simulink model "BMS"  (R2022b)
settings: Solver=VariableStepAuto  StartTime=0.0  StopTime=inf  RelTol=1e-3
libraries: simulink x2
settings Model: PacingRate=0.710000  Creator=admin  LastModifiedBy=DELL

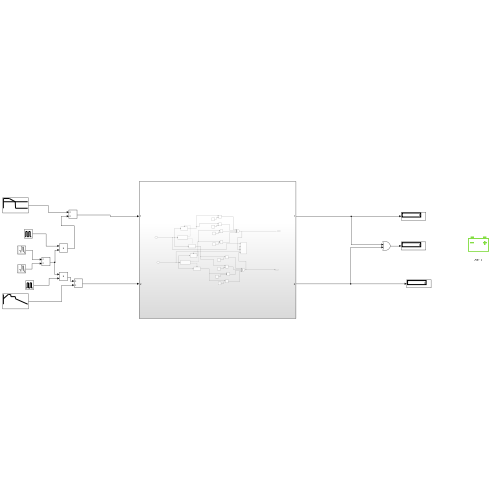
[thumbnail: Simulink's stored preview of the top-level diagram]
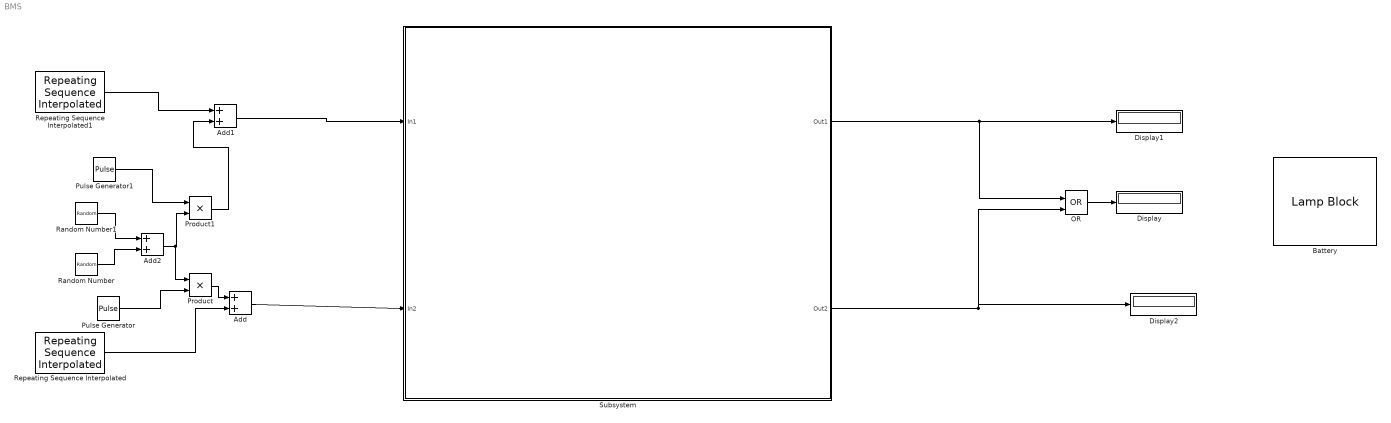
== system BMS ==
  Add : Sum
  Add1 : Sum
  Add2 : Sum
  Battery : LampBlock  LabelPosition=Bottom  Icon=Battery
  Display : Display
  Display1 : Display
  Display2 : Display
  OR : Logic  Operator=OR  IconShape=distinctive  AllPortsSameDT=off  OutDataTypeStr=boolean
  Product : Product
  Product1 : Product
  Pulse Generator : DiscretePulseGenerator  PulseType=Time based  Period=22  PulseWidth=2  PhaseDelay=20
  Pulse Generator1 : DiscretePulseGenerator  PulseType=Time based  Period=37  PulseWidth=2  PhaseDelay=40
  Random Number : RandomNumber  Variance=7  SampleTime=0.1
  Random Number1 : RandomNumber  Mean=-5  Variance=13  SampleTime=0.1
  Repeating Sequence Interpolated : simulink/Sources/Repeating Sequence Interpolated  OutValues=[12.8 14.2 14.2 13.5 13.5 12.8 11].'  TimeValues=[0 0.2 0.30 0.31 0.49 0.50 1].'  LookUpMeth=Interpolation-Use End Values  tsamp=0.01  OutMin=[]  OutMax=[]  OutDataTypeStr=double  OutputDataTypeScalingMode=double  OutDataType=fixdt(0,8)  OutScaling=2^-10
  Repeating Sequence Interpolated1 : simulink/Sources/Repeating Sequence Interpolated  OutValues=[3 3 0 -6 -6].'  TimeValues=[0 0.25 0.49 0.5 1].'  LookUpMeth=Interpolation-Use End Values  tsamp=0.01  OutMin=[]  OutMax=[]  OutDataTypeStr=double  OutputDataTypeScalingMode=double  OutDataType=fixdt(0,8)  OutScaling=2^-10
  Subsystem : Subsystem
  wires:
  Pulse Generator/1 -> Product/2
  Pulse Generator1/1 -> Product1/1
  Random Number/1 -> Add2/2
  Add2/1 -> Product/1, Product1/2
  Random Number1/1 -> Add2/1
  Product1/1 -> Add1/2
  Repeating Sequence Interpolated1/1 -> Add1/1
  Product/1 -> Add/1
  Repeating Sequence Interpolated/1 -> Add/2
  OR/1 -> Display/1
  Add1/1 -> Subsystem/1(In1)
  Add/1 -> Subsystem/2(In2)
  Subsystem/1(Out1) -> OR/1, Display1/1
  Subsystem/2(Out2) -> OR/2, Display2/1

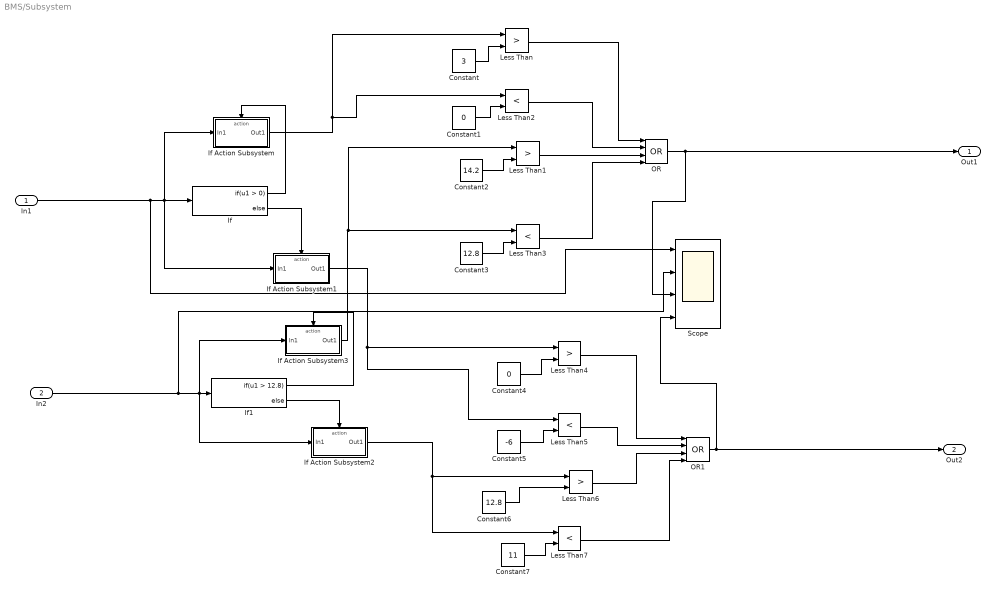
== system BMS/Subsystem ==
  In1 : Inport
  In2 : Inport  Port=2
  Constant : Constant  Value=3
  Constant1 : Constant  Value=0
  Constant2 : Constant  Value=14.2
  Constant3 : Constant  Value=12.8
  Constant4 : Constant  Value=0
  Constant5 : Constant  Value=-6
  Constant6 : Constant  Value=12.8
  Constant7 : Constant  Value=11
  If : If
  If Action Subsystem : Subsystem  TreatAsAtomicUnit=on
  If Action Subsystem1 : Subsystem  TreatAsAtomicUnit=on
  If Action Subsystem2 : Subsystem  TreatAsAtomicUnit=on
  If Action Subsystem3 : Subsystem  TreatAsAtomicUnit=on
  If1 : If  IfExpression=u1 > 12.8
  Less Than{,1,4,6} (4 alike) : RelationalOperator  Operator=>  OutDataTypeStr=boolean  RndMeth=Simplest  InputSameDT=off
  Less Than{2..3,5,7} (4 alike) : RelationalOperator  Operator=<  OutDataTypeStr=boolean  RndMeth=Simplest  InputSameDT=off
  OR : Logic  Operator=OR  Inputs=4  IconShape=distinctive  AllPortsSameDT=off  OutDataTypeStr=boolean
  OR1 : Logic  Operator=OR  Inputs=4  IconShape=distinctive  AllPortsSameDT=off  OutDataTypeStr=boolean
  Scope : Scope  NumInputPorts=4
  Out1 : Outport
  Out2 : Outport  Port=2
  wires:
  Constant4/1 -> Less Than4/2
  Constant6/1 -> Less Than6/2
  In1/1 -> Scope/1, If Action Subsystem1/1(In1), If/1, If Action Subsystem/1(In1)
  If Action Subsystem1/1(Out1) -> Less Than5/1, Less Than4/1
  If1/1 -> If Action Subsystem3/Action
  Constant7/1 -> Less Than7/2
  Less Than1/1 -> OR/3
  Less Than4/1 -> OR1/1
  If Action Subsystem3/1(Out1) -> Less Than1/1, Less Than3/1
  Constant/1 -> Less Than/2
  OR/1 -> Out1/1, Scope/3
  Constant1/1 -> Less Than2/2
  Constant5/1 -> Less Than5/2
  Constant2/1 -> Less Than1/2
  If/2 -> If Action Subsystem1/Action
  Less Than2/1 -> OR/2
  In2/1 -> Scope/2, If Action Subsystem3/1(In1), If Action Subsystem2/1(In1), If1/1
  Constant3/1 -> Less Than3/2
  Less Than7/1 -> OR1/4
  Less Than3/1 -> OR/4
  If1/2 -> If Action Subsystem2/Action
  Less Than5/1 -> OR1/2
  Less Than/1 -> OR/1
  If Action Subsystem/1(Out1) -> Less Than/1, Less Than2/1
  OR1/1 -> Out2/1, Scope/4
  Less Than6/1 -> OR1/3
  If/1 -> If Action Subsystem/Action
  If Action Subsystem2/1(Out1) -> Less Than7/1, Less Than6/1

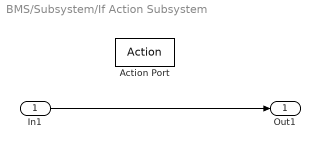
== system BMS/Subsystem/If Action Subsystem ==
  In1 : Inport
  Action Port : ActionPort  ActionPortLabel=if(u1 > 0)
  Out1 : Outport
  wires:
  In1/1 -> Out1/1

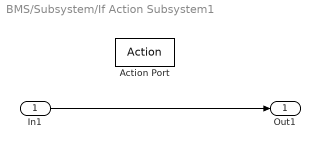
== system BMS/Subsystem/If Action Subsystem1 ==
  In1 : Inport
  Action Port : ActionPort  ActionPortLabel=else
  Out1 : Outport
  wires:
  In1/1 -> Out1/1

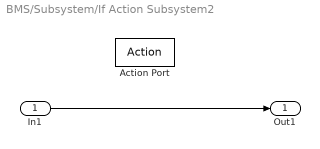
== system BMS/Subsystem/If Action Subsystem2 ==
  In1 : Inport
  Action Port : ActionPort  ActionPortLabel=else
  Out1 : Outport
  wires:
  In1/1 -> Out1/1

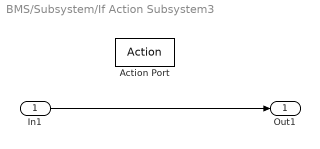
== system BMS/Subsystem/If Action Subsystem3 ==
  In1 : Inport
  Action Port : ActionPort  ActionPortLabel=if(u1 > 12.8)
  Out1 : Outport
  wires:
  In1/1 -> Out1/1
